simulink model "F4PhantomRunningModel"  (R2023b)
settings: Solver=ode4  StartTime=0.0  StopTime=t_final  FixedStep=Ts  RelTol=1e-3
values from neighbouring files (symbols this model uses):
  alpha1 = 2.6    [F4ModelCode.m]    (also in F4ModelCodeV2.m; F4ModelCodeV2Q2PartD.m; F4PhantomModelCode.m)
  Hw3Coeffs = [c_L_alpha c_L_delta_E c_L_i_H c_m_alpha c_m_delta_E c_m_i_H c_L_alphadot c_L_q c_m_alphadot c_m_q c_D_alpha]    [F4ModelCode.m]    (also in F4ModelCodeV2.m; F4ModelCodeV2Q2PartD.m; F4PhantomModelCode.m = [c_L_alpha c_L_delta_E c_L_i_H c_m_alpha c_m_delta_E c_m_i_H)
  Hw4Coeffs = [c_Y_beta c_Y_delta_A c_Y_delta_R c_n_beta c_n_delta_A c_n_delta_R c_l_beta c_l_delta_A c_l_delta_R c_l_p c_Y_p c_n_p c_l_r c_Y_r c_n_r]    [F4ModelCode.m]    (also in F4ModelCodeV2.m; F4ModelCodeV2Q2PartD.m; F4PhantomModelCode.m)
  i_H_vector = horzcat(timeVec,i_H)    [F4ModelCode.m]    (also in F4ModelCodeV2.m; F4ModelCodeV2Q2PartD.m)
  InitialInputs = [qbar1 S_ft2 c_D_1 c_L_1 cbar_ft c_m_1 uv b_ft alphadot]    [F4ModelCode.m]    (also in F4ModelCodeV2.m; F4ModelCodeV2Q2PartD.m)
  uCoeffs = [c_L_u c_D_u c_m_u]    [F4ModelCode.m]    (also in F4ModelCodeV2.m; F4ModelCodeV2Q2PartD.m; F4PhantomModelCode.m = [c_L_u c_D_u])
  uk = [c_D_delta_E c_D_q c_D_i_H c_Y_1 c_Y_betadot c_l_betadot c_n_1 c_n_betadot]    [F4ModelCode.m]    (also in F4ModelCodeV2.m; F4ModelCodeV2Q2PartD.m)
libraries: shared6dof x1
settings Model: Creator=Owner  LastModifiedBy=Owner
settings DataIOCC: ReturnWorkspaceOutputs=off
settings DebuggingCC: UnconnectedInputMsg=warning  UnconnectedOutputMsg=warning  UnconnectedLineMsg=warning
settings HardwareCC: ProdHWDeviceType=AMD->x86-64 (Windows64)
settings ModelReferenceCC: EnableRefExpFcnMdlSchedulingChecks=on

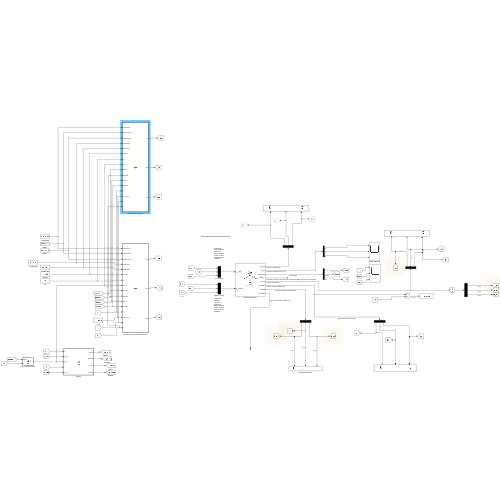
[thumbnail: Simulink's stored preview of the top-level diagram]
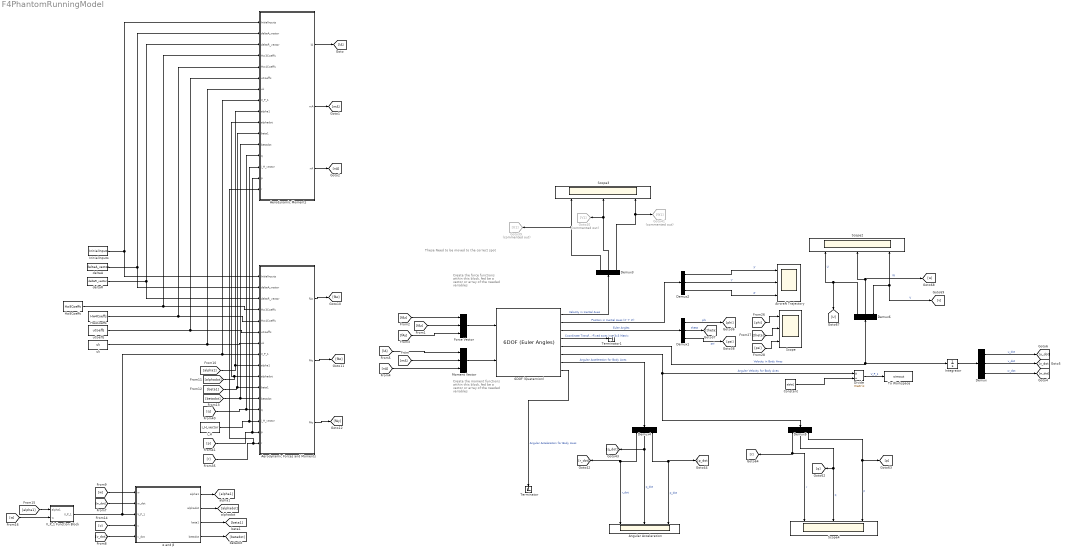
== system F4PhantomRunningModel ==
  note: These Need to be moved to the correct spot
  note: Create the moment functions within this block, fed be a vector or array of the needed variables
  note: Create the force functions within this block, fed be a vector or array of the needed variables
  6DOF (Quaternion) : shared6dof/6DOF (Euler Angles)  units=English (Velocity in ft/s)  mtype=Fixed  rep=Quaternion  xme_0=InitialInertialPosition  Vm_0=InitialVelocity  eul_0=InitialEulerOrientation  pm_0=InitialRotationRates  mass_0=1.0  mass_e=0.5  mass_f=2.0  inertia=eye(3)  inertia_e=eye(3)  inertia_f=2*eye(3)  k_quat=1.0  vre_flag=on  abi_flag=off  aMode=0  xme_statename=''  Vm_statename=''  eul_statename=''  quat_statename=''  pm_statename=''  mass_statename=''
      settings: LibrarySourceBlock=aerolib6dof2/6DOF (Quaternion)
  Aerodynamic Forces and Moments : MATLAB Function  TreatAsAtomicUnit=on
  Aerodynamic Moments : MATLAB Function  TreatAsAtomicUnit=on
  Aircraft Trajectory : Scope  NumInputPorts=3
  Angular Acceleration : Scope  NumInputPorts=3
  Constant : Constant  Value=alpha1
  Demux{,1..6} (7 alike) : Demux  Outputs=3
  Divide : Product  Inputs=*/  Multiplication=Matrix(*)
  Force Vector : Mux  Inputs=3
  Goto39 : Goto  Commented=on  GotoTag=U1
  Goto40 : Goto  Commented=on  GotoTag=V1
  Goto41 : Goto  Commented=on  GotoTag=W1
  Hw3Coeffs : Constant  Value=Hw3Coeffs
  Hw4Coeffs : Constant  Value=Hw4Coeffs
  InitialInputs : Constant  Value=InitialInputs
  Integrator : Integrator
  Moment Vector : Mux  Inputs=3
  Scope{,2..4} (4 alike) : Scope  NumInputPorts=3
  Terminator : Terminator
  Terminator1 : Terminator
  To Workspace : ToWorkspace  VariableName=simout  SaveFormat=Timeseries  SampleTime=-1
  V_P_1 Function Block : MATLAB Function  TreatAsAtomicUnit=on
  "deltaA " : FromWorkspace  VariableName=deltaA_vector  OutDataTypeStr=double
  "deltaR " : FromWorkspace  VariableName=deltaR_vector  OutDataTypeStr=double
  i_H : Constant  Value=i_H_vector
  uCoeffs : Constant  Value=uCoeffs
  uk : Constant  Value=uk
  α and β : MATLAB Function  TreatAsAtomicUnit=on
  wires:
  Force Vector/1 -> 6DOF (Quaternion)/1
  6DOF (Quaternion)/1 -> Demux3/1  "Velocity in Inertial Axes"
  6DOF (Quaternion)/2 -> Demux2/1  "Position in Inertial Axes (X' Y' Z')"
  6DOF (Quaternion)/3 -> Demux1/1  "Euler Angles"
  6DOF (Quaternion)/4 -> Terminator1/1  "Coordinate Transformation from Flat Earth axes to Body-Fixed axes in a 3x3 Matrix"
  6DOF (Quaternion)/5 -> Integrator/1, Demux6/1  "Velocity in Body Axes"
  6DOF (Quaternion)/6 -> Demux5/1, Divide/1  "Angular Velocity for Body Axes"
  6DOF (Quaternion)/7 -> Demux4/1  "Angular Acceleration for Body Axes"
  6DOF (Quaternion)/8 -> Terminator/1  "Angular Acceleration for Body Axes"
  Aerodynamic Forces and Moments/1(fAx) -> [fAx]
  Aerodynamic Forces and Moments/2(fAz) -> [fAz]
  Aerodynamic Forces and Moments/3(fAy) -> [fAy]
  Moment Vector/1 -> 6DOF (Quaternion)/2
  [fAz] -> Force Vector/2
  [fAx] -> Force Vector/1
  [mA] -> Moment Vector/2
  [fAy] -> Force Vector/3
  [nA] -> Moment Vector/3
  [lA] -> Moment Vector/1
  Demux1/1 -> [phi]  "phi"
  Demux1/2 -> [theta]  "theta"
  Demux1/3 -> [psi]  "psi"
  [phi] -> Scope/1
  [theta] -> Scope/2
  [psi] -> Scope/3
  Demux2/1 -> Aircraft Trajectory/1  "X'"
  Demux2/2 -> Aircraft Trajectory/2  "Y'"
  Demux2/3 -> Aircraft Trajectory/3  "Z'"
  Demux3/1 -> Scope3/1, Goto39/1
  Demux3/2 -> Goto40/1, Scope3/2
  Demux3/3 -> Scope3/3, Goto41/1
  Demux4/1 -> [r_dot], Angular Acceleration/1  "r_dot"
  Demux4/2 -> [q_dot], Angular Acceleration/2  "q_dot"
  Demux4/3 -> [p_dot], Angular Acceleration/3  "p_dot"
  Demux5/1 -> [r], Scope4/1  "r"
  Demux5/2 -> [q], Scope4/2  "q"
  Demux5/3 -> [p], Scope4/3  "p"
  Constant/1 -> Divide/2
  Divide/1 -> To Workspace/1  "V_P_1"
  [p] -> Aerodynamic Moments/15(p), Aerodynamic Forces and Moments/15(p)
  [r] -> Aerodynamic Moments/16(r), Aerodynamic Forces and Moments/16(r)
  α and β/1(alpha1) -> [alpha1]
  α and β/4(betadot) -> [betadot]
  α and β/3(beta1) -> [beta1]
  α and β/2(alphadot) -> [alphadot]
  Demux6/3 -> [v], Scope2/3  "V"
  Demux6/2 -> [w], Scope2/2  "W"
  Demux6/1 -> Scope2/1, [U]  "U"
  [q] -> Aerodynamic Moments/13(q), Aerodynamic Forces and Moments/13(q)
  InitialInputs/1 -> Aerodynamic Moments/1(InitialInputs), Aerodynamic Forces and Moments/1(InitialInputs)
  "deltaA "/1 -> Aerodynamic Moments/2(deltaA_vector), Aerodynamic Forces and Moments/2(deltaA_vector)
  Hw3Coeffs/1 -> Aerodynamic Moments/4(Hw3Coeffs), Aerodynamic Forces and Moments/4(Hw3Coeffs)
  Hw4Coeffs/1 -> Aerodynamic Moments/5(Hw4Coeffs), Aerodynamic Forces and Moments/5(Hw4Coeffs)
  uCoeffs/1 -> Aerodynamic Moments/6(uCoeffs), Aerodynamic Forces and Moments/6(uCoeffs)
  uk/1 -> Aerodynamic Moments/7(uk), Aerodynamic Forces and Moments/7(uk)
  i_H/1 -> Aerodynamic Moments/14(i_H_vector), Aerodynamic Forces and Moments/14(i_H_vector)
  [alpha1] -> Aerodynamic Forces and Moments/9(alpha1), Aerodynamic Moments/9(alpha1)
  [alphadot] -> Aerodynamic Forces and Moments/10(alphadot), Aerodynamic Moments/10(alphadot)
  [beta1] -> Aerodynamic Forces and Moments/11(beta1), Aerodynamic Moments/11(beta1)
  [betadot] -> Aerodynamic Forces and Moments/12(betadot), Aerodynamic Moments/12(betadot)
  Integrator/1 -> Demux/1
  Demux/1 -> [u_dot]  "u_dot"
  Demux/2 -> [v_dot]  "v_dot"
  Demux/3 -> [w_dot]  "w_dot"
  [w_dot] -> α and β/2(w_dot)
  [v_dot] -> α and β/5(v_dot)
  [w] -> α and β/1(w)
  [v] -> α and β/4(v)
  V_P_1 Function Block/1(V_P_1) -> Aerodynamic Moments/8(V_P_1), Aerodynamic Forces and Moments/8(V_P_1), α and β/3(V_P_1)
  [alpha1] -> V_P_1 Function Block/1(alpha1)
  [w] -> V_P_1 Function Block/2(w)
  "deltaR "/1 -> Aerodynamic Moments/3(deltaR_vector), Aerodynamic Forces and Moments/3(deltaR_vector)
  Aerodynamic Moments/1(lA) -> [lA]
  Aerodynamic Moments/2(mA) -> [mA]
  Aerodynamic Moments/3(nA) -> [nA]

== matlab function F4PhantomRunningModel/Aerodynamic Forces and Moments ==
  data: InitialInputs input; deltaA_vector input; deltaR_vector input; Hw3Coeffs input; Hw4Coeffs input; uCoeffs input; uk input; V_P_1 input; alpha1 input; alphadot input; beta1 input; betadot input; q input; i_H_vector input; fAx output; fAz output; fAy output; p input; r input
function [ fAx, fAz,  fAy]  = fcn(InitialInputs, deltaA_vector, deltaR_vector, Hw3Coeffs, Hw4Coeffs, uCoeffs, uk, V_P_1, alpha1, alphadot, beta1, betadot, q, i_H_vector, p, r)
qbar1 = InitialInputs(1); S_ft2 = InitialInputs(2); c_D_1 = InitialInputs(3); c_L_1 = InitialInputs(4); cbar_ft = InitialInputs(5); c_m_1 = InitialInputs(6); uv = InitialInputs(7); b_ft = InitialInputs(8);
% deltaA_vector = CSv(1); deltaR_vector = CSv(2); deltaS_vector = CSv(3); 
% deltaA = CSc(1); deltaS = CSc(2); deltaR = CSc(3);
c_L_alpha = Hw3Coeffs(1); c_L_delta_E = Hw3Coeffs(2); c_L_i_H = Hw3Coeffs(3); c_m_alpha = Hw3Coeffs(4); c_m_delta_E = Hw3Coeffs(5); c_m_i_H = Hw3Coeffs(6); c_L_alphadot = Hw3Coeffs(7); c_L_q = Hw3Coeffs(8); c_m_alphadot = Hw3Coeffs(9); c_m_q = Hw3Coeffs(10); c_D_alpha = Hw3Coeffs(11);
c_Y_beta = Hw4Coeffs(1); c_Y_delta_A = Hw4Coeffs(2); c_Y_delta_R = Hw4Coeffs(3); c_n_beta = Hw4Coeffs(4); c_n_delta_A = Hw4Coeffs(5); c_n_delta_R = Hw4Coeffs(6); c_l_beta = Hw4Coeffs(7); c_l_delta_A = Hw4Coeffs(8); c_l_delta_R = Hw4Coeffs(9); c_l_p = Hw4Coeffs(10); c_Y_p = Hw4Coeffs(11); c_n_p = Hw4Coeffs(12); c_l_r = Hw4Coeffs(13); c_Y_r = Hw4Coeffs(14); c_n_r = Hw4Coeffs(15);
c_L_u = uCoeffs(1); c_D_u = uCoeffs(2); c_m_u = uCoeffs(3); 
c_D_delta_E = uk(1);  c_D_q = uk(2); c_D_i_H = uk(3); c_Y_1 = uk(4); c_Y_betadot = uk(5); c_l_betadot = uk(6); c_n_1 = uk(7); c_n_betadot = uk(8);

deltaE = 0;

%FAx = -qbar1*S_ft2*c_D_1;
fAx = (qbar1*S_ft2)*(((-(c_D_u+(2*c_D_1)))*(uv/V_P_1)) + ((c_D_alpha + c_L_1)*(alpha1)) - c_D_alpha*((alphadot*cbar_ft)/(2*V_P_1)) - c_D_q*((q*cbar_ft)/(2*V_P_1)) - (c_D_delta_E*deltaE)-(c_D_i_H*i_H_vector));

%FAz = -qbar1*S_ft2*c_L_1;
fAz = (qbar1*S_ft2)*(((-(c_L_u+(2*c_L_1)))*(uv/V_P_1)) + ((c_L_alpha + c_D_1)*(alpha1)) - c_L_alphadot*((alphadot*cbar_ft)/(2*V_P_1)) - c_L_q*((q*cbar_ft)/(2*V_P_1)) - (c_L_delta_E*deltaE)-(c_L_i_H*i_H_vector));

%FAy = -qbar1*S_ft2*c_Y_1;
fAy = -qbar1*S_ft2 * ((c_Y_beta*beta1) + c_Y_betadot * ((betadot*b_ft)/(2*V_P_1)) + c_Y_p*((p*b_ft)/(2*V_P_1)) + c_Y_r * ((r*b_ft)/(2*V_P_1)) +(c_Y_delta_A * deltaA_vector) + (c_Y_delta_R*deltaR_vector));

%LA = -qbar1*S_ft2*b_ft*c_L_1;
% lA = -qbar1*S_ft2*b_ft*((c_l_beta*beta1) + c_l_betadot * ((betadot*b_ft)/(2*V_P_1)) + c_l_p*((p*b_ft)/(2*V_P_1)) + c_l_r * ((r*b_ft)/(2*V_P_1)) +(c_l_delta_A * deltaA_vector) + (c_l_delta_R*deltaR_vector));
% 
% %MA = -qbar1*S_ft2*cbar_ft*c_m_1; %%%%This line is throwing an error
% mA = (qbar1*S_ft2*cbar_ft)*(((-(c_m_u+(2*c_m_1)))*(uv/V_P_1)) + (c_m_alpha*alpha1) + c_m_alphadot*((alphadot*cbar_ft)/(2*V_P_1)) + c_m_q*((q*cbar_ft)/(2*V_P_1)) + (c_m_delta_E*deltaE)+(c_L_i_H*i_H_vector));
% 
% %NA = -qbar1*S_ft2*b_ft*c_n_1;
% nA = -qbar1*S_ft2*b_ft*((c_n_beta*beta1) + c_n_betadot * ((betadot*b_ft)/(2*V_P_1)) + c_n_p*((p*b_ft)/(2*V_P_1)) + c_n_r * ((r*b_ft)/(2*V_P_1)) +(c_n_delta_A * deltaA_vector) + (c_n_delta_R*deltaR_vector));

%Need to get rid of fAy and lA and nA, leave MA and mA

== matlab function F4PhantomRunningModel/α and β ==
  data: w input; alpha1 output; alphadot output; beta1 output; w_dot input; V_P_1 input; v input; v_dot input; betadot output
function [alpha1, alphadot, beta1, betadot] = fcn(w, w_dot, V_P_1, v, v_dot)

alpha1 = w/V_P_1;

alphadot = w_dot/V_P_1;

beta1 = v/V_P_1;

betadot = v_dot/V_P_1;

== matlab function F4PhantomRunningModel/V_P_1 Function Block ==
  data: alpha1 input; V_P_1 output; w input
function V_P_1 = fcn(alpha1,w)

alpha1 = deg2rad(alpha1); 
V_P_1 = w/alpha1;

== matlab function F4PhantomRunningModel/Aerodynamic Moments ==
  data: InitialInputs input; deltaA_vector input; deltaR_vector input; Hw3Coeffs input; Hw4Coeffs input; uCoeffs input; uk input; V_P_1 input; alpha1 input; alphadot input; beta1 input; betadot input; q input; i_H_vector input; lA output; mA output; nA output; p input; r input
function [lA,  mA, nA]  = fcn(InitialInputs, deltaA_vector, deltaR_vector, Hw3Coeffs, Hw4Coeffs, uCoeffs, uk, V_P_1, alpha1, alphadot, beta1, betadot, q, i_H_vector, p, r)
qbar1 = InitialInputs(1); S_ft2 = InitialInputs(2); c_D_1 = InitialInputs(3); c_L_1 = InitialInputs(4); cbar_ft = InitialInputs(5); c_m_1 = InitialInputs(6); uv = InitialInputs(7); b_ft = InitialInputs(8);
% deltaA_vector = CSv(1); deltaR_vector = CSv(2); deltaS_vector = CSv(3); 
% deltaA = CSc(1); deltaS = CSc(2); deltaR = CSc(3);
c_L_alpha = Hw3Coeffs(1); c_L_delta_E = Hw3Coeffs(2); c_L_i_H = Hw3Coeffs(3); c_m_alpha = Hw3Coeffs(4); c_m_delta_E = Hw3Coeffs(5); c_m_i_H = Hw3Coeffs(6); c_L_alphadot = Hw3Coeffs(7); c_L_q = Hw3Coeffs(8); c_m_alphadot = Hw3Coeffs(9); c_m_q = Hw3Coeffs(10); c_D_alpha = Hw3Coeffs(11);
c_Y_beta = Hw4Coeffs(1); c_Y_delta_A = Hw4Coeffs(2); c_Y_delta_R = Hw4Coeffs(3); c_n_beta = Hw4Coeffs(4); c_n_delta_A = Hw4Coeffs(5); c_n_delta_R = Hw4Coeffs(6); c_l_beta = Hw4Coeffs(7); c_l_delta_A = Hw4Coeffs(8); c_l_delta_R = Hw4Coeffs(9); c_l_p = Hw4Coeffs(10); c_Y_p = Hw4Coeffs(11); c_n_p = Hw4Coeffs(12); c_l_r = Hw4Coeffs(13); c_Y_r = Hw4Coeffs(14); c_n_r = Hw4Coeffs(15);
c_L_u = uCoeffs(1); c_D_u = uCoeffs(2); c_m_u = uCoeffs(3); 
c_D_delta_E = uk(1);  c_D_q = uk(2); c_D_i_H = uk(3); c_Y_1 = uk(4); c_Y_betadot = uk(5); c_l_betadot = uk(6); c_n_1 = uk(7); c_n_betadot = uk(8);

deltaE = 0;

% %FAx = -qbar1*S_ft2*c_D_1;
% fAx = (qbar1*S_ft2)*(((-(c_D_u+(2*c_D_1)))*(uv/V_P_1)) + ((c_D_alpha + c_L_1)*(alpha1)) - c_D_alpha*((alphadot*cbar_ft)/(2*V_P_1)) - c_D_q*((q*cbar_ft)/(2*V_P_1)) - (c_D_delta_E*deltaE)-(c_D_i_H*i_H_vector));
% 
% %FAz = -qbar1*S_ft2*c_L_1;
% fAz = (qbar1*S_ft2)*(((-(c_L_u+(2*c_L_1)))*(uv/V_P_1)) + ((c_L_alpha + c_D_1)*(alpha1)) - c_L_alphadot*((alphadot*cbar_ft)/(2*V_P_1)) - c_L_q*((q*cbar_ft)/(2*V_P_1)) - (c_L_delta_E*deltaE)-(c_L_i_H*i_H_vector));
% 
% %FAy = -qbar1*S_ft2*c_Y_1;
% fAy = -qbar1*S_ft2 * ((c_Y_beta*beta1) + c_Y_betadot * ((betadot*b_ft)/(2*V_P_1)) + c_Y_p*((p*b_ft)/(2*V_P_1)) + c_Y_r * ((r*b_ft)/(2*V_P_1)) +(c_Y_delta_A * deltaA_vector) + (c_Y_delta_R*deltaR_vector));

%LA = -qbar1*S_ft2*b_ft*c_L_1;
lA = -qbar1*S_ft2*b_ft*((c_l_beta*beta1) + c_l_betadot * ((betadot*b_ft)/(2*V_P_1)) + c_l_p*((p*b_ft)/(2*V_P_1)) + c_l_r * ((r*b_ft)/(2*V_P_1)) +(c_l_delta_A * deltaA_vector) + (c_l_delta_R*deltaR_vector));
% 
% %MA = -qbar1*S_ft2*cbar_ft*c_m_1; %%%%This line is throwing an error
mA = (qbar1*S_ft2*cbar_ft)*(((-(c_m_u+(2*c_m_1)))*(uv/V_P_1)) + (c_m_alpha*alpha1) + c_m_alphadot*((alphadot*cbar_ft)/(2*V_P_1)) + c_m_q*((q*cbar_ft)/(2*V_P_1)) + (c_m_delta_E*deltaE)+(c_L_i_H*i_H_vector));
% 
% %NA = -qbar1*S_ft2*b_ft*c_n_1;
nA = -qbar1*S_ft2*b_ft*((c_n_beta*beta1) + c_n_betadot * ((betadot*b_ft)/(2*V_P_1)) + c_n_p*((p*b_ft)/(2*V_P_1)) + c_n_r * ((r*b_ft)/(2*V_P_1)) +(c_n_delta_A * deltaA_vector) + (c_n_delta_R*deltaR_vector));

%Need to get rid of fAy and lA and nA, leave MA and mA
